simulink subsystem "OriginalLoadsEstimator"  (R2024b)
settings: Solver=VariableStepAuto  StartTime=0.0  StopTime=10.0  RelTol=1e-3
settings Model: Creator=jhummel  LastModifiedBy=jhummel
settings ModelReferenceCC: EnableRefExpFcnMdlSchedulingChecks=on
settings RTWCC: GPUComputeCapability=3.5

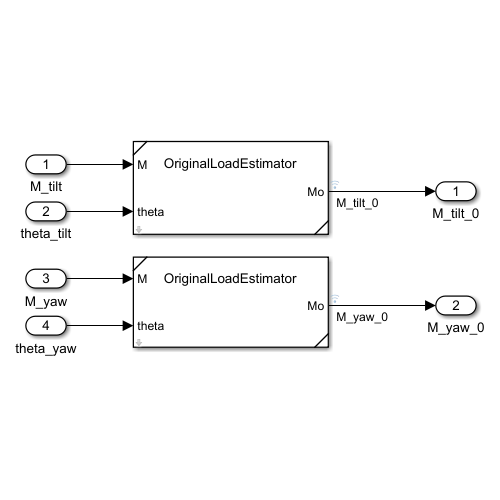
[thumbnail: Simulink's stored preview of the top-level diagram]
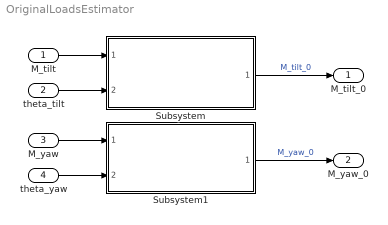
== system OriginalLoadsEstimator ==
  M_tilt : Inport
  theta_tilt : Inport  Port=2
  M_yaw : Inport  Port=3
  theta_yaw : Inport  Port=4
  Subsystem : Subsystem  ReferencedSubsystem=OriginalLoadEstimator  w=w_originalLoadEstimator  dMdTheta=dMtdThetat
  Subsystem1 : Subsystem  ReferencedSubsystem=OriginalLoadEstimator  w=w_originalLoadEstimator  dMdTheta=dMydThetay
  M_tilt_0 : Outport
  M_yaw_0 : Outport  Port=2
  wires:
  theta_tilt/1 -> Subsystem/2
  M_yaw/1 -> Subsystem1/1
  M_tilt/1 -> Subsystem/1
  Subsystem/1 -> M_tilt_0/1  "M_tilt_0"
  Subsystem1/1 -> M_yaw_0/1  "M_yaw_0"
  theta_yaw/1 -> Subsystem1/2
